simulink model "LinearActiveSuspension"  (R2018b)
settings: Solver=VariableStepAuto  StartTime=0.0  StopTime=tmax  FixedStep=0.001  RelTol=1e-3
values from neighbouring files (symbols this model uses):
  A = [  0       1         0          -1 ... (first row only)    [load_params.m]
  B = [    0        0 ... (first row only)    [load_params.m]
  C = [   1      0     0     0 ... (first row only)    [load_params.m]
  D = [ 0   0 ... (first row only)    [load_params.m]
undefined symbols (not defined in the file or in its folder): i
settings Model: Creator=alexj  LastModifiedBy=alexj

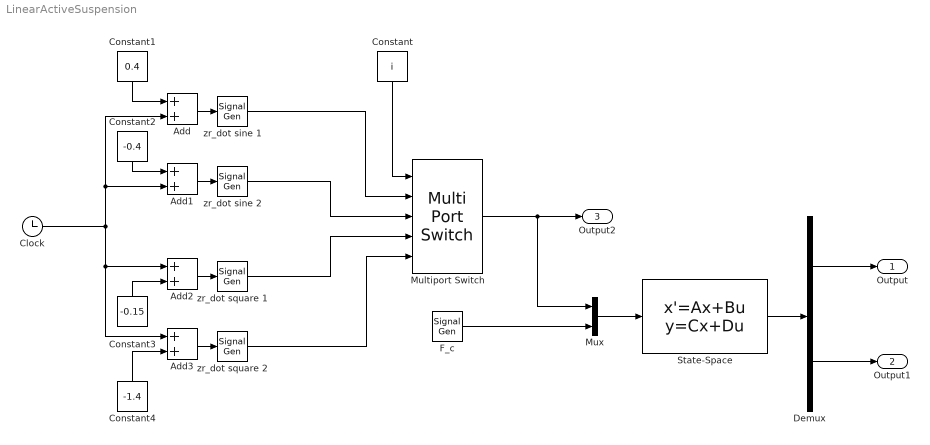
== system LinearActiveSuspension ==
  Add{,1..3} (4 alike) : Sum
  Clock : Clock
  Constant : Constant  Value=i
  Constant1 : Constant  Value=0.4
  Constant2 : Constant  Value=-0.4
  Constant3 : Constant  Value=-0.15
  Constant4 : Constant  Value=-1.4
  Demux : Demux  Outputs=2
  F_c : SignalGenerator  Amplitude=0  Units=rad/sec
  Multiport Switch : MultiPortSwitch  Inputs=4
  Mux : Mux  Inputs=2
  State-Space : StateSpace  A=A  B=B  C=C  D=D  InitialCondition=[0 0 0 0]  ContinuousStateAttributes="\"\""
  zr_dot sine 1 : SignalGenerator  TimeSource=Use external signal  Amplitude=0.015  Frequency=0.5
  zr_dot sine 2 : SignalGenerator  TimeSource=Use external signal  Amplitude=0.015  Frequency=0.5
  zr_dot square 1 : SignalGenerator  WaveForm=square  TimeSource=Use external signal  Amplitude=0.01  Frequency=0.2
  zr_dot square 2 : SignalGenerator  WaveForm=square  TimeSource=Use external signal  Amplitude=0.005  Frequency=0.2
  Output : Outport  SignalName=suspension_travel
  Output1 : Outport  Port=2  SignalName=body_acc
  Output2 : Outport  Port=3  SignalName=zr_dot
  wires:
  Mux/1 -> State-Space/1
  State-Space/1 -> Demux/1
  Demux/1 -> Output/1
  Demux/2 -> Output1/1
  F_c/1 -> Mux/2
  Add/1 -> zr_dot sine 1/1
  Multiport Switch/1 -> Output2/1, Mux/1
  Constant/1 -> Multiport Switch/1
  zr_dot sine 1/1 -> Multiport Switch/2
  zr_dot sine 2/1 -> Multiport Switch/3
  zr_dot square 1/1 -> Multiport Switch/4
  zr_dot square 2/1 -> Multiport Switch/5
  Constant1/1 -> Add/1
  Clock/1 -> Add3/1, Add2/1, Add1/2, Add/2
  Add1/1 -> zr_dot sine 2/1
  Add3/1 -> zr_dot square 2/1
  Add2/1 -> zr_dot square 1/1
  Constant2/1 -> Add1/1
  Constant3/1 -> Add2/2
  Constant4/1 -> Add3/2
